simulink model "Problem_5"  (R2020b)
settings: Solver=VariableStepAuto  StartTime=0.0  StopTime=10.0  RelTol=1e-3
InitFcn:
  | R=10;
  | C=10e-5;
settings Model: Creator=Lenovo  LastModifiedBy=Lenovo

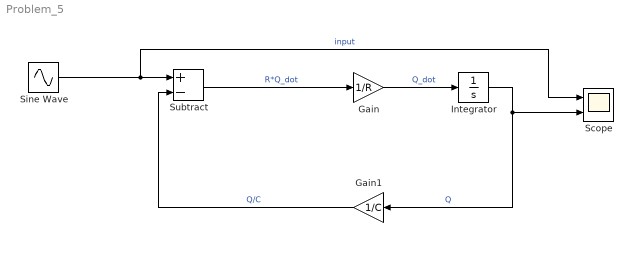
== system Problem_5 ==
  Gain : Gain  Gain=1/R
  Gain1 : Gain  Gain=1/C
  Integrator : Integrator  InitialCondition=1
  Scope : Scope  NumInputPorts=2
  Sine Wave : Sin  SampleTime=0
  Subtract : Sum  Inputs=+-
  wires:
  Subtract/1 -> Gain/1  "R*Q_dot"
  Gain/1 -> Integrator/1  "Q_dot"
  Sine Wave/1 -> Scope/1, Subtract/1  "input"
  Integrator/1 -> Scope/2, Gain1/1  "Q"
  Gain1/1 -> Subtract/2  "Q/C"
